simulink model "DCC_DTC_v1"  (R2023b)
settings: Solver=FixedStepDiscrete  StartTime=0.0  StopTime=0.4  MaxStep=1e-  RelTol=1e-6
undefined symbols (not defined in the file): DiscIntNeverNeededParam
libraries: spsDCVoltageSourceLib x1, spsGroundLib x1, spsPermanentMagnetSynchronousMachineLib x1, simulink x1, spsThreePhaseVIMeasurementLib x1, spsUniversalBridgeLib x1, sps_lib x1
settings Model: Creator=rainy  LastModifiedBy=rainy
settings DataIOCC: ReturnWorkspaceOutputs=off

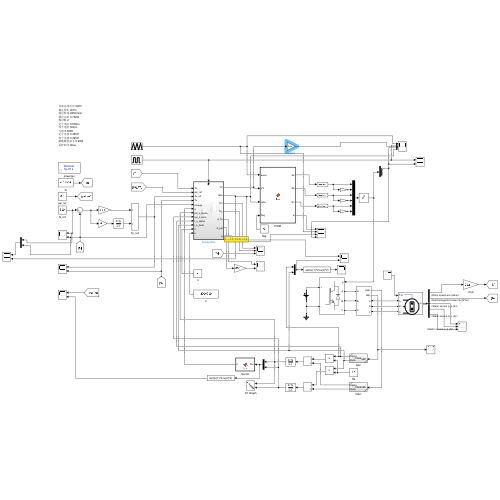
[thumbnail: Simulink's stored preview of the top-level diagram]
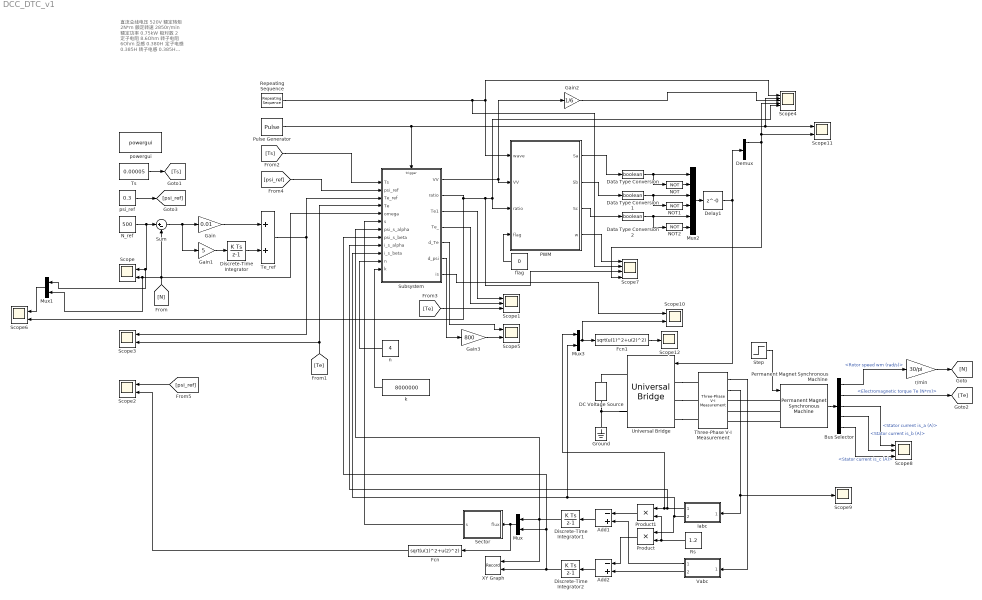
== system DCC_DTC_v1 ==
  note: 直流总线电压 520V
      | 额定转矩 2N*m
      | 额定转速 2850r/min
      | 额定功率 0.75kW
      | 极对数 2
      | 定子电阻 8.6Ohm
      | 转子电阻 6Ohm
      | 互感 0.380H
      | 定子电感 0.385H
      | 转子电感 0.385H
      | 磁链幅值参考 0.9Wb
      | 采样时间 80us
  Add1 : Sum  Inputs=-+
  Add2 : Sum  Inputs=-+
  Bus Selector : BusSelector  OutputSignals=Rotor speed wm (rad/s),Electromagnetic torque Te (N*m),Stator current is_a (A),Stator current is_b (A),Stator current is_c (A)
  DC Voltage Source : spsDCVoltageSourceLib/DC Voltage Source  Amplitude=311  Measurements=Voltage
  Data Type Conversion : DataTypeConversion  OutDataTypeStr=boolean  SaturateOnIntegerOverflow=off  RndMeth=Floor
  Data Type Conversion1 : DataTypeConversion  OutDataTypeStr=boolean  SaturateOnIntegerOverflow=off  RndMeth=Floor
  Data Type Conversion2 : DataTypeConversion  OutDataTypeStr=boolean  SaturateOnIntegerOverflow=off  RndMeth=Floor
  Delay1 : Delay  DelayLength=0  SampleTime=0.000001
  Demux : Demux  Outputs=6
  Discrete-Time Integrator : DiscreteIntegrator  SampleTime=-1  ICPrevOutput=DiscIntNeverNeededParam  ICPrevScaledInput=DiscIntNeverNeededParam
  Discrete-Time Integrator1 : DiscreteIntegrator  SampleTime=-1  ICPrevOutput=DiscIntNeverNeededParam  ICPrevScaledInput=DiscIntNeverNeededParam
  Discrete-Time Integrator2 : DiscreteIntegrator  SampleTime=-1  ICPrevOutput=DiscIntNeverNeededParam  ICPrevScaledInput=DiscIntNeverNeededParam
  Fcn : Fcn  Expr=sqrt(u(1)^2+u(2)^2)
  Fcn1 : Fcn  Expr=sqrt(u(1)^2+u(2)^2)
  Gain : Gain  Gain=0.01
  Gain1 : Gain  Gain=5
  Gain2 : Gain  Gain=1/6
  Gain3 : Gain  Gain=800
  Ground : spsGroundLib/Ground  LConnTagsString=a
  Iabc : Subsystem  ReferencedSubsystem=Clark
  Mux : Mux  Inputs=2
  Mux1 : Mux  Inputs=2
  Mux2 : Mux  Inputs=6
  Mux3 : Mux  Inputs=2
  NOT : Logic  Operator=NOT  IconShape=distinctive  AllPortsSameDT=off  OutDataTypeStr=boolean
  NOT1 : Logic  Operator=NOT  IconShape=distinctive  AllPortsSameDT=off  OutDataTypeStr=boolean
  NOT2 : Logic  Operator=NOT  IconShape=distinctive  AllPortsSameDT=off  OutDataTypeStr=boolean
  N_ref : Constant  Value=500
  PWM : MATLAB Function  TreatAsAtomicUnit=on
  Permanent Magnet Synchronous Machine : spsPermanentMagnetSynchronousMachineLib/Permanent Magnet Synchronous Machine  NbPhases=3  FluxDistribution=Sinusoidal  RotorType=Round  MechanicalLoad=Torque Tm  PresetModel=No  ShowDetailedParameters=on  MeasurementBus=off  Resistance=1.2  Inductance=8.5e-3  dqInductances=[8.5e-3,8.5e-3]  La=0.0085  MachineConstant=Flux linkage established by magnets (V.s)  Flux=0.175  VoltageCst=126.966  TorqueCst=1.05  Flat=120  Mechanical=[0.0008 0.0004924 4 0]  PolePairs=4  InitialConditions=[0 0 0 0]  InitialConditions5ph=[0 0 0 0 0 0]  RefAngle=Aligned with phase A axis (original Park)  IterativeDiscreteModel=Trapezoidal non iterative  TsBlock=-1  TsPowergui=0
  Product : Product
  Product1 : Product
  Pulse Generator : DiscretePulseGenerator  PulseType=Time based  Period=0.00005
  Repeating Sequence : simulink/Sources/Repeating Sequence  rep_seq_t=[0 0.000025 0.00005]  rep_seq_y=[0 1 0]
  Rs : Constant  Value=1.2
  Scope{,2..3,5..6,10..11} (7 alike) : Scope  NumInputPorts=2
  Scope1 : Scope  NumInputPorts=3
  Scope12 : Scope
  Scope4 : Scope  NumInputPorts=5
  Scope7 : Scope  NumInputPorts=4
  Scope8 : Scope  NumInputPorts=3
  Scope9 : Scope
  Sector : MATLAB Function  TreatAsAtomicUnit=on
  Step : Step  Time=0.02  SampleTime=0
  Subsystem : Subsystem
  Sum : Sum  Inputs=|+-
  Te_ref : Sum
  Three-Phase V-I Measurement : spsThreePhaseVIMeasurementLib/Three-Phase V-I Measurement  VoltageMeasurement=phase-to-ground  SetLabelV=off  LabelV=Vabc  Vpu=off  VpuLL=off  CurrentMeasurement=yes  SetLabelI=off  LabelI=Iabc  Ipu=off  Pbase=100e6  Vbase=500e3  OutputType=Complex  PhasorSimulation=off  PSBequivalent=0
  Ts : Constant  Value=0.00005
  Universal Bridge : spsUniversalBridgeLib/Universal Bridge  Arms=3  SnubberResistance=1e5  SnubberCapacitance=inf  Device=IGBT / Diodes  Ron=1e-3  Lon=0  ForwardVoltages="[  0  0  ]"  ForwardVoltage=0  GTOparameters=[ 10e-6 , 20e-6 ]  IGBTparameters=[ 1e-6 , 2e-6 ]  Measurements=None  Measurements_2=None  converterType=Rectifier
  Vabc : Subsystem  ReferencedSubsystem=Clark
  XY Graph : Record  FileSettingsInternal="{\"entries\":[{\"content\":{\"excelSettings\":{\"content\":{},\"type\":\"Streamout.ExcelSettings\"}},\"type\":\"Streamout.FileSettingStorage\",\"uuid\":\"\"}],\"packageUris\":[\"http:\\/\\/schema.mathworks.com\\/mf0\\/streamout_blocks\\/R2020a\"],\"version\":\"1.0\"}"  Layout=[1 1]  SignalsInternal="{\"entries\":[{\"content\":{\"signals\":[{\"content\":{\"blockPath\":[],\"dimensions\":[1],\"domain\":\"\",\"lineColor\":\"#a2142f\",\"plots\":[1],\"port\":1,\"sid\":[\"\"],\"signalID\":4121,\"signalName\":\"Discrete-Time\\nIntegrator1\"},\"type\":\"RecordBlkView.Signal\",\"uuid\":\"\"},{\"content\":{\"blockPath\":[],\"dimensions\":[1],\"domain\":\"\",\"lineColor\":\"#139fff\",\"plots\":[1],\"port\":2,\"sid\":[\"\"],\"signalID\":4125,\"signalName\":\"Discrete-Time\\nIntegrator2\"},\"type\":\"RecordBlkView.Signal\",\"uuid\":\"\"}]},\"type\":\"RecordBlkView.InputSignals\",\"uuid\":\"\"}],\"packageUris\":[\"http:\\/\\/schema.mathworks.com\\/mf0\\/streamout_blocks\\/R2020a\"],\"version\":\"1.0\"}"  VisualizationBindings="{\"xyplotplugin\":{\"info\":[{\"series\":[{\"bindingParametersList\":[{\"parameter\":\"X-Axis\",\"signalID\":4121,\"signalName\":\"Discrete-Time\\nIntegrator1\"},{\"parameter\":\"Y-Axis\",\"signalID\":4125,\"signalName\":\"Discrete-Time\\nIntegrator2\"}],\"seriesID\":2107}],\"subplotID\":1}]}}"  CompatibilityTag=XY  st=-1
  flag : Constant  Value=0
  k : Constant  Value=8000000
  n : Constant  Value=4
  powergui : sps_lib/powergui  Priority=1  SimulationMode=Discrete  SampleTime=5e-7  frequency=60  Iterations=50  frequencyindice=0  Pbase=100e6  ErrMax=1e-4  UnitsV=kV  UnitsW=MW  buscounter=0  FunctionMessages=off  echomessages=off  EnableUseOfTLC=off  CurrentSourceSwitches=off  DisableSnubberDevices=off  DisableRonSwitches=off  DisableVfSwitches=off  DisplayEquations=off  AutomaticDiscreteSolvers=off  SolverType=Tustin/Backward Euler (TBE)  Interpol=off  ExternalGateDelay=off  methode=off  Ts=100  x0status=blocks  SPID=on  SwTol=0  HookPort=off  NonlinearTolerance=1e-4  nMaxIteration=100  ContinueOnMaxIteration=off  RestoreLinks=warning  ResistiveCurrentMeasurement=off  Frange=[0:2:500]  Ylog=off  Xlog=on  ShowGrid=off  save=off  variable=ZData  structure=0  ZoomFFT=off  StartTime=0.0  cycles=1  DisplayStyle=1  fundamental=60  FreqAxis=off  MaxFrequency=1000  frequencyindicesteady=1  RmsSteady=1  display=off
  psi_ref : Constant  Value=0.3
  r/min : Gain  Gain=30/pi
  wires:
  N_ref/1 -> Mux1/1, Scope/1, Sum/1
  Sum/1 -> Gain/1, Gain1/1
  Gain1/1 -> Discrete-Time Integrator/1
  Gain/1 -> Te_ref/1
  Permanent Magnet Synchronous Machine/1 -> Bus Selector/1
  Bus Selector/1 -> r/min/1  "<Rotor speed wm (rad/s)>"
  r/min/1 -> [N]
  [N] -> Subsystem/5(omega), Mux1/2, Scope/2, Sum/2
  NOT1/1 -> Mux2/4
  Data Type Conversion2/1 -> NOT2/1, Mux2/5
  NOT2/1 -> Mux2/6
  Data Type Conversion/1 -> NOT/1, Mux2/1
  NOT/1 -> Mux2/2
  Data Type Conversion1/1 -> NOT1/1, Mux2/3
  Iabc/1 -> Mux3/1, Product1/1, Subsystem/9(i_s_alpha)
  Iabc/2 -> Mux3/2, Subsystem/10(i_s_beta), Product/1
  Rs/1 -> Product/2, Product1/2
  Product1/1 -> Add1/1
  Vabc/1 -> Add1/2
  Product/1 -> Add2/1
  Vabc/2 -> Add2/2
  Add2/1 -> Discrete-Time Integrator2/1
  Add1/1 -> Discrete-Time Integrator1/1
  Ts/1 -> [Ts]
  Discrete-Time Integrator1/1 -> Subsystem/7(psi_s_alpha), XY Graph/1, Mux/1
  Discrete-Time Integrator2/1 -> XY Graph/2, Subsystem/8(psi_s_beta), Mux/2
  Mux/1 -> Fcn/1, Sector/1(flux)
  Te_ref/1 -> Subsystem/3(Te_ref), Scope3/1
  Bus Selector/2 -> [Te]  "<Electromagnetic torque Te (N*m)>"
  [Te] -> Scope3/2, Subsystem/4(Te)
  Three-Phase V-I Measurement/2 -> Iabc/1, Scope9/1
  Three-Phase V-I Measurement/1 -> Vabc/1
  Discrete-Time Integrator/1 -> Te_ref/2
  [Te] -> Scope1/3
  psi_ref/1 -> [psi_ref]
  [psi_ref] -> Scope2/1
  Fcn/1 -> Scope2/2
  PWM/3(Sc) -> Data Type Conversion2/1
  PWM/2(Sb) -> Data Type Conversion1/1
  PWM/1(Sa) -> Data Type Conversion/1
  Delay1/1 -> Demux/1, Universal Bridge/1
  [Ts] -> Subsystem/1(Ts)
  [psi_ref] -> Subsystem/2(psi_ref)
  Sector/1(s) -> Subsystem/6(s)
  Subsystem/1(VV) -> PWM/2(VV), Gain2/1
  Subsystem/2(ratio) -> Scope6/2, Scope7/3, Scope4/5, PWM/3(ratio)
  Subsystem/3(Te1) -> Scope1/1
  Subsystem/4(Te_) -> Scope1/2
  Repeating Sequence/1 -> Scope7/2, Scope4/1, PWM/1(wave)
  Pulse Generator/1 -> Scope11/1, Scope4/2, Subsystem/Trigger
  Mux2/1 -> Delay1/1
  Demux/1 -> Scope11/2, Scope4/4, Scope7/4
  Gain2/1 -> Scope4/3
  n/1 -> Subsystem/11(n)
  k/1 -> Subsystem/12(k)
  Subsystem/5(d_Te) -> Scope5/1
  Subsystem/6(d_psi) -> Gain3/1
  Gain3/1 -> Scope5/2
  flag/1 -> PWM/4(flag)
  Mux1/1 -> Scope6/1
  PWM/4(w) -> Scope7/1
  Bus Selector/3 -> Scope8/1  "<Stator current is_a (A)>"
  Bus Selector/4 -> Scope8/2  "<Stator current is_b (A)>"
  Bus Selector/5 -> Scope8/3  "<Stator current is_c (A)>"
  Step/1 -> Permanent Magnet Synchronous Machine/1
  Subsystem/7(is) -> Scope10/1
  Mux3/1 -> Fcn1/1, Scope10/2
  Fcn1/1 -> Scope12/1
  connections:
  Universal Bridge/RConn2 -- Ground/LConn1 -- DC Voltage Source/LConn1
  Permanent Magnet Synchronous Machine/LConn2 -- Three-Phase V-I Measurement/RConn2
  Permanent Magnet Synchronous Machine/LConn1 -- Three-Phase V-I Measurement/RConn1
  Universal Bridge/LConn3 -- Three-Phase V-I Measurement/LConn3
  Universal Bridge/LConn1 -- Three-Phase V-I Measurement/LConn1
  Universal Bridge/LConn2 -- Three-Phase V-I Measurement/LConn2
  DC Voltage Source/RConn1 -- Universal Bridge/RConn1
  Permanent Magnet Synchronous Machine/LConn3 -- Three-Phase V-I Measurement/RConn3

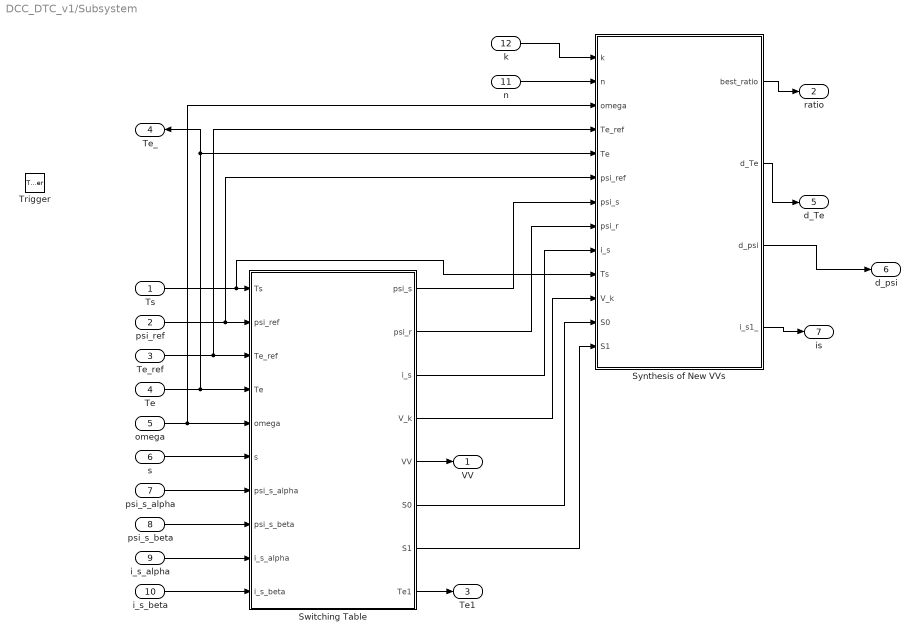
== system DCC_DTC_v1/Subsystem ==
  Ts : Inport
  psi_ref : Inport  Port=2
  Te_ref : Inport  Port=3
  Te : Inport  Port=4
  omega : Inport  Port=5
  s : Inport  Port=6
  psi_s_alpha : Inport  Port=7
  psi_s_beta : Inport  Port=8
  i_s_alpha : Inport  Port=9
  i_s_beta : Inport  Port=10
  n : Inport  Port=11
  k : Inport  Port=12
  Trigger : TriggerPort  VariantControl=(inherit)  PortDimensions=1
  Switching Table : MATLAB Function  TreatAsAtomicUnit=on
  Synthesis of New VVs : MATLAB Function  TreatAsAtomicUnit=on
  VV : Outport
  ratio : Outport  Port=2
  Te1 : Outport  Port=3
  Te_ : Outport  Port=4  VectorParamsAs1DForOutWhenUnconnected=off
  d_Te : Outport  Port=5
  d_psi : Outport  Port=6
  is : Outport  Port=7
  wires:
  n/1 -> Synthesis of New VVs/2(n)
  Switching Table/5(VV) -> VV/1
  psi_s_beta/1 -> Switching Table/8(psi_s_beta)
  Ts/1 -> Synthesis of New VVs/10(Ts), Switching Table/1(Ts)
  Switching Table/7(S1) -> Synthesis of New VVs/13(S1)
  s/1 -> Switching Table/6(s)
  Switching Table/6(S0) -> Synthesis of New VVs/12(S0)
  psi_ref/1 -> Switching Table/2(psi_ref), Synthesis of New VVs/6(psi_ref)
  i_s_alpha/1 -> Switching Table/9(i_s_alpha)
  omega/1 -> Synthesis of New VVs/3(omega), Switching Table/5(omega)
  Te_ref/1 -> Synthesis of New VVs/4(Te_ref), Switching Table/3(Te_ref)
  i_s_beta/1 -> Switching Table/10(i_s_beta)
  psi_s_alpha/1 -> Switching Table/7(psi_s_alpha)
  Te/1 -> Te_/1, Synthesis of New VVs/5(Te), Switching Table/4(Te)
  Switching Table/8(Te1) -> Te1/1
  Synthesis of New VVs/1(best_ratio) -> ratio/1
  Switching Table/1(psi_s) -> Synthesis of New VVs/7(psi_s)
  Switching Table/4(V_k) -> Synthesis of New VVs/11(V_k)
  Switching Table/3(i_s) -> Synthesis of New VVs/9(i_s)
  Switching Table/2(psi_r) -> Synthesis of New VVs/8(psi_r)
  k/1 -> Synthesis of New VVs/1(k)
  Synthesis of New VVs/2(d_Te) -> d_Te/1
  Synthesis of New VVs/3(d_psi) -> d_psi/1
  Synthesis of New VVs/4(i_s1_) -> is/1

== matlab function DCC_DTC_v1/Sector ==
  data: flux input; s output
function s = fcn(flux)

% 将\psi_{\aplha}和\psi_{\beta}分解为三相
a1 = flux(1);
b1 = flux(1)*(-0.5) + sqrt(3)/2*flux(2);
c1 = flux(1)*(-0.5) - sqrt(3)/2*flux(2);

% a1 > 0，有扇区126
% b1 > 0，有扇区234
% c1 > 0，有扇区456
% n为a1 b1 c1中>0的个数，0 < n < 3
% 
% a b c | s
%-------|---
% 1 1 0 | 2
% 1 0 1 | 6
% 1 0 0 | 1
% 0 1 1 | 4
% 0 1 0 | 3
% 0 0 1 | 5

if(flux(2) == 0)
    N = 4;
else
    if(a1 > 0)
        a = 1;
    else
        a = 0;
    end
    
    if(b1 > 0)
        b = 1;
    else
        b = 0;
    end
    
    if(c1 > 0)
        c = 1;
    else
        c = 0;
    end
    
    N = 4*a+2*b+c;
end

if(N==0 || N==7)
    N = 4;
end

Sector_table=[5 3 4 1 6 2];

s = Sector_table(N);

== matlab function DCC_DTC_v1/Subsystem/Switching Table ==
  data: psi_s output; psi_r output; i_s output; V_k output; Ts input; psi_ref input; Te_ref input; Te input; VV output; S0 output; S1 output; omega input; s input; psi_s_alpha input; psi_s_beta input; i_s_alpha input; i_s_beta input; Te1 output
function [psi_s, psi_r, i_s, V_k, VV, S0, S1, Te1] = fcn(Ts, psi_ref, Te_ref, Te, omega, s, psi_s_alpha, psi_s_beta, i_s_alpha, i_s_beta)

% 给定的参数值
P = 4; % 极对数
R_s = 1.2; % 定子电阻
R_r = 1.2; % 转子电阻
L_m = 0.008; % 磁链互感
L_s = 0.0085; % 定子电感
L_r = 0.0085; % 转子电感
sigma = 1-L_m^2/(L_s*L_r);
V = 311;

psi_s = psi_s_alpha + 1i*psi_s_beta;
i_s = i_s_alpha + 1i*i_s_beta;
psi_r = L_r/L_m*psi_s + i_s*(L_m - L_s*L_r/L_m);


% 计算 S0
S0 = 1.5 * P/2 * L_m/(sigma * L_s * L_r) * ...
    (-((R_s/(sigma * L_s) + R_r/(sigma * L_r)) * imag(psi_r' * psi_s) - omega * real(psi_r' * psi_s)));


Te1 = Te + Ts*S0;
psi = sqrt(psi_s_alpha^2 +psi_s_beta^2);

if(Te_ref > Te)
    if(psi_ref > psi)
        VV = s+1;
    else
        VV = s+2;
    end
else
    if(psi_ref > psi)
        VV = s-1;
    else
        VV = s-2;
    end
end

if(VV < 1)
    VV = VV+6;
end
if(VV > 6)
    VV = VV-6;
end

V_k = cos(pi/6*(VV-1))*V + 1i*sin(pi/6*(VV-1))*V;
S1 = S0 + 1.5 * P/2 * L_m/(sigma * L_s * L_r) * imag(psi_r' * V_k);

== matlab function DCC_DTC_v1/Subsystem/Synthesis of New VVs ==
  data: k input; n input; omega input; Te_ref input; Te input; psi_ref input; psi_s input; psi_r input; i_s input; Ts input; V_k input; best_ratio output; S0 input; S1 input; d_Te output; d_psi output; i_s1_ output
function [best_ratio, d_Te, d_psi, i_s1_]  = fcn(k, n, omega, Te_ref, Te, psi_ref, psi_s, psi_r, i_s, Ts, V_k, S0, S1)

R_s = 1.2; % 定子电阻
R_r = 1.2; % 转子电阻
L_m = 0.008; % 磁链互感
L_s = 0.0085; % 定子电感
L_r = 0.0085; % 转子电感
sigma = 1-L_m^2/(L_s*L_r);
V = 311;

persistent flag V_s
if isempty(flag)
    flag = 1;
    V_s = 0 + 1i*0;
end

k_r = L_m/L_r;
R_sigma = R_s + k_r^2 * R_r;
tau_r = L_r / R_r;
tau_sigma = sigma * L_s / R_sigma;
i_s1 = (1 - Ts/tau_sigma)*i_s + Ts/tau_sigma * (1/R_sigma * ((k_r / tau_r - 1i * k_r * omega) * psi_r + V_s));
i_s1_ = i_s1;

g_min = 200000;
best_ratio = 1;
d_Te = 0;
d_psi = 0;

for i=1:n+1
    ratio = (i-1)*1/n;

    Te1 = Te + Ts*ratio*S1 + Ts*(1-ratio)*S0;
    psi1 = psi_s + Ts*ratio*V_k - R_s*Ts*i_s1;
    
    d_Te = abs(Te_ref - Te1);
    d_psi = abs(psi_ref - abs(psi1));

    g = d_Te + k*d_psi;

    if(g < g_min)
        g_min = g;
        best_ratio =ratio;
    end
end
best_ratio
V_s = V_k;

== matlab function DCC_DTC_v1/PWM ==
  data: wave input; VV input; ratio input; Sa output; Sb output; Sc output; flag input; w output
function [Sa, Sb, Sc, w] = fcn(wave, VV, ratio, flag)

sw = [1 0 0; 1 1 0; 0 1 0; 0 1 1; 0 0 1; 1 0 1];

if(VV<1 || VV>6)
    VV = 1;
end

if(wave >= 1 - ratio || flag == 0)
    Sa= sw(VV, 1);
    Sb= sw(VV, 2);
    Sc= sw(VV, 3);
    w = 1;
else
    Sa = 0;
    Sb = 0;
    Sc = 0;
    w = 0;
end
